simulink model "ECO_RM_WEC_EGEC"  (R2025a)
settings: Solver=ode4  StartTime=0  StopTime=120  FixedStep=0.00025  MaxStep=0.00025  RelTol=1e-3
values from neighbouring files (symbols this model uses):
  r = 0.043    [wecSimInputFile.m]
  simu = simulationClass()    [wecSimInputFile.m]
undefined symbols (not defined in the file or in its folder): body, constraint, DiscIntNeverNeededParam, geometry, hydroData, pto, ptoSim
libraries: WECSim_Lib_Body_Elements x2, WECSim_Lib_Frames x1, WECSim_Lib_Constraints x1, WECSim_Lib_PTOs x1
settings Model: Creator=pam1061  LastModifiedBy=pam1061
settings SolverCC: ZeroCrossControl=DisableAll  AutoInsertRateTranBlk=on
settings DataIOCC: ReturnWorkspaceOutputs=off
settings OptimizationCC: SimCompilerOptimization=on

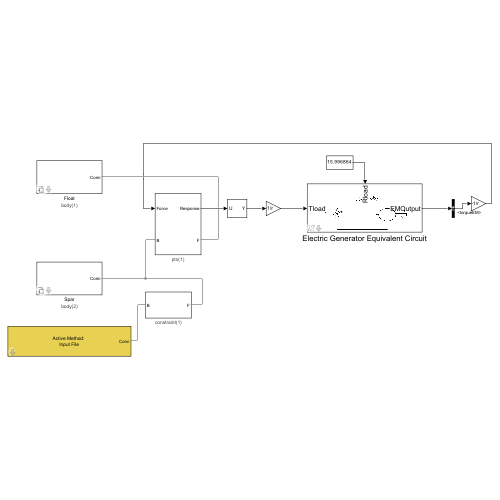
[thumbnail: Simulink's stored preview of the top-level diagram]
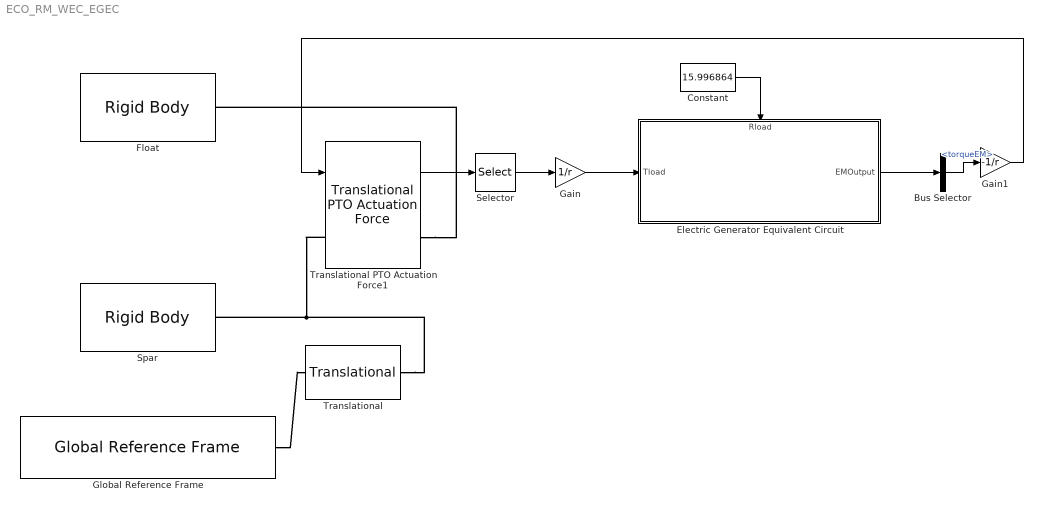
== system ECO_RM_WEC_EGEC ==
  Bus Selector : BusSelector  OutputSignals=torqueEM
  Constant : Constant  Value=15.996864
  Electric Generator Equivalent Circuit : Subsystem  AncestorBlock=WECSim_Lib_PTOSim/Electric/Electric Generator Equivalent Circuit  mask{ptoSim=ptoSim(1), InputFiletext=Use WEC-Sim input file to define Electric Machine parameters, Ra=0.890000, La=0.00500000, Ke=4.106198, bShaft=0, Jem=5.422000e-03}
      mask prompts: ptoSim "Electric Machine Name"; Ra "Armature Resistance [ohm]"; La "Armature Inductance [H]"; Ke "Back-emf or Torque constant [V/(rad/s)]"; bShaft "Rotor Damping [N s/m]"; Jem "Rotor Inertia [kg m^2]"
      mask init:
      | if exist('ptoSim','var')
      |     h=[gcb '/To Workspace'];
      |     responseName=['ptoSim' num2str(ptoSim.number) '_out'];
      |     set_param(h,'VariableName',responseName);
      | end
      | clear h responseName
      settings: PortSchema="{\"entries\":[{\"content\":{\"sides\":[{\"content\":{\"connectorIds\":[\"In1\"]},\"type\":\"ConnectorPlacement.EquallySpacedRectSide\",\"uuid\":\"38b15b7d-d952-45b6-9eb0-5d473736364e\"},{\"content\":{\"connectorIds\":[\"Out1\"],\"side\":\"RIGHT\"},\"type\":\"ConnectorPlacement.EquallySpacedRectSide\",\"uuid\":\"de64adb9-f2de-4dd5-b519-c63af884483d\"},{\"content\":{\"connectorIds\":[\"In2\"],\"side\":\"TOP\"},\"type\":\"ConnectorPlacement.EquallySpacedRectSide\",\"uuid\":\"eaa9506a-5e37-41b4-975c-a8d526700d36\"},{\"content\":{\"connectorIds\":[],\"side\":\"HIDDEN\"},\"type\":\"ConnectorPlacement.EquallySpacedRectSide\",\"uuid\":\"f8da1221-e5bc-4844-b966-beaaa1d6bf60\"}]},\"type\":\"ConnectorPlacement.EquallySpacedConnector\",\"uuid\":\"4da2b473-e94d-42dc-9143-64fbcbf5d9e1\"}],\"packageUris\":[\"http://schema.mathworks.com/mf0/Connector/R2020b\"],\"version\":\"1.0\"}"
      mask DialogControl CustomParameterGroup Prompt: Custom Parameters
      mask DialogControl EMParameters Prompt: Electric Machine Parameters
      mask Display: image('ElectricMotor.png'); % Use "Edit Image" on toolstrip to change.
  Float : WECSim_Lib_Body_Elements/Rigid Body  body=body(1)  h5File=hydroData/*.h5  geometryFile=geometry/*.stl  mass=0  inertia=0 0 0  inertiaProducts=0 0 0  nonHydro=0  nonlinearHydro=0  centerGravity=0 0 0  centerBuoyancy=0 0 0  dof=6  volume=0  displacement=0 0 0  axis=0 1 0  angle=0  option=0  cd=0 0 0  ca=0 0 0  area=0 0 0  VME=0  rgME=0 0 0  z=0 0 1
  Gain : Gain  Gain=1/r
  Gain1 : Gain  Gain=-1/r
  Global Reference Frame : WECSim_Lib_Frames/Global Reference Frame  waves=waves  simu=simu  InputMethod=Input File  InputFile=wecSimInputFile.m  mode=normal  explorer=off  solver=ode4  startTime=0  rampTime=100  endTime=400  dt=0.1  cicEndTime=60  stateSpace=0  WaveClass=regular  height=2.5  period=8  elevationFile=NOT DEFINED  spectrumFile=NOT DEFINED  direction=0  spread=1  spectrumType=NOT DEFINED  phaseSeed=0  option=EqualEnergy
  Selector : Selector  InputPortWidth=18  IndexOptions=Index vector (dialog)  Indices=9  OutputSizes=1
  Spar : WECSim_Lib_Body_Elements/Rigid Body  body=body(2)  h5File=hydroData/*.h5  geometryFile=geometry/*.stl  mass=0  inertia=0 0 0  inertiaProducts=0 0 0  nonHydro=0  nonlinearHydro=0  centerGravity=0 0 0  centerBuoyancy=0 0 0  dof=6  volume=0  displacement=0 0 0  axis=0 1 0  angle=0  option=0  cd=0 0 0  ca=0 0 0  area=0 0 0  VME=0  rgME=0 0 0  z=0 0 1
  Translational : WECSim_Lib_Constraints/Translational  constraint=constraint(1)  loc="0  0  0"  displacement=0 0 0  y=0 1 0  z=0 0 1  upperLimitSpecify=off  upperLimitBound=0  upperLimitTransitionRegionWidth=0  upperLimitStiffness=0  upperLimitDamping=0  lowerLimitSpecify=off  lowerLimitBound=0  lowerLimitTransitionRegionWidth=0  lowerLimitStiffness=0  lowerLimitDamping=0
      settings: AttributesFormatString=%<constraint>
  Translational PTO Actuation Force1 : WECSim_Lib_PTOs/Translational PTO Actuation Force  pto=pto(1)  loc="0  0  0"  stiffness=0  damping=0  equilibriumPosition=0  pretension=0  displacement=0 0 0  y=0 1 0  z=0 0 1  upperLimitSpecify=off  upperLimitBound=0  upperLimitTransitionRegionWidth=0  upperLimitStiffness=0  upperLimitDamping=0  lowerLimitSpecify=off  lowerLimitBound=0  lowerLimitTransitionRegionWidth=0  lowerLimitStiffness=0  lowerLimitDamping=0
      settings: AttributesFormatString=%<pto>
  wires:
  Translational PTO Actuation Force1/1 -> Selector/1
  Gain1/1 -> Translational PTO Actuation Force1/1
  Constant/1 -> Electric Generator Equivalent Circuit/2(Rload)
  Selector/1 -> Gain/1
  Gain/1 -> Electric Generator Equivalent Circuit/1(Tload)
  Electric Generator Equivalent Circuit/1(EMOutput) -> Bus Selector/1
  Bus Selector/1 -> Gain1/1  "<torqueEM>"
  connections:
  Global Reference Frame/RConn1 -- Translational/LConn1
  Translational/RConn1 -- Translational PTO Actuation Force1/LConn1 -- Spar/RConn1
  Translational PTO Actuation Force1/RConn1 -- Float/RConn1

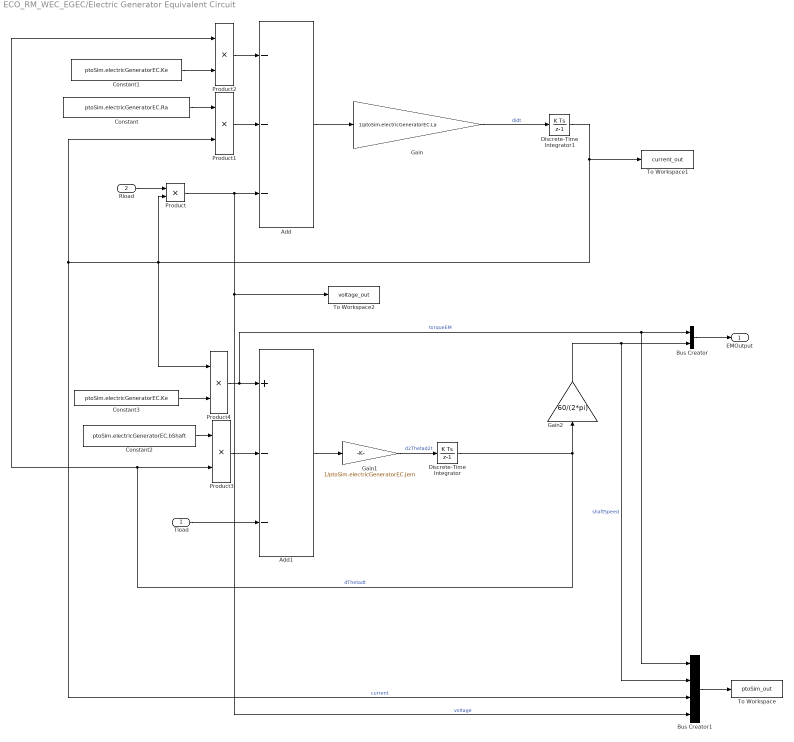
== system ECO_RM_WEC_EGEC/Electric Generator Equivalent Circuit ==
  Tload : Inport
  Rload : Inport  Port=2
  Add : Sum  Inputs=---
  Add1 : Sum  Inputs=+--
  Bus Creator : BusCreator  Inputs=2
  Bus Creator1 : BusCreator  Inputs=4
  Constant : Constant  Value=ptoSim.electricGeneratorEC.Ra
  Constant1 : Constant  Value=ptoSim.electricGeneratorEC.Ke
  Constant2 : Constant  Value=ptoSim.electricGeneratorEC.bShaft
  Constant3 : Constant  Value=ptoSim.electricGeneratorEC.Ke
  Discrete-Time Integrator : DiscreteIntegrator  InitialCondition=(2*pi/60)*ptoSim.electricGeneratorEC.wShaftIni  SampleTime=-1  ICPrevOutput=DiscIntNeverNeededParam  ICPrevScaledInput=DiscIntNeverNeededParam
  Discrete-Time Integrator1 : DiscreteIntegrator  InitialCondition=ptoSim.electricGeneratorEC.currentIni  SampleTime=-1  ICPrevOutput=DiscIntNeverNeededParam  ICPrevScaledInput=DiscIntNeverNeededParam
  Gain : Gain  Gain=1/ptoSim.electricGeneratorEC.La
  Gain1 : Gain  Gain=1/ptoSim.electricGeneratorEC.Jem
  Gain2 : Gain  Gain=60/(2*pi)
  Product{,1..4} (5 alike) : Product
  To Workspace : ToWorkspace  VariableName=ptoSim_out  SaveFormat=Structure With Time  SampleTime=simu.dtOut
  To Workspace1 : ToWorkspace  VariableName=current_out  SampleTime=-1
  To Workspace2 : ToWorkspace  VariableName=voltage_out  SampleTime=-1
  EMOutput : Outport
  wires:
  Bus Creator1/1 -> To Workspace/1
  Gain2/1 -> Bus Creator/2, Bus Creator1/2  "shaftSpeed"
  Bus Creator/1 -> EMOutput/1
  Constant3/1 -> Product4/2
  Product4/1 -> Add1/1, Bus Creator/1, Bus Creator1/1  "torqueEM"
  Discrete-Time Integrator/1 -> Gain2/1, Product3/2, Product2/1  "dThetadt"
  Constant2/1 -> Product3/1
  Product3/1 -> Add1/2
  Gain1/1 -> Discrete-Time Integrator/1  "d2Thetad2t"
  Add1/1 -> Gain1/1
  Tload/1 -> Add1/3
  Constant1/1 -> Product2/2
  Product2/1 -> Add/1
  Constant/1 -> Product1/1
  Product1/1 -> Add/2
  Product/1 -> Add/3, To Workspace2/1, Bus Creator1/4  "voltage"
  Discrete-Time Integrator1/1 -> To Workspace1/1, Product1/2, Bus Creator1/3, Product/2, Product4/1  "current"
  Rload/1 -> Product/1
  Gain/1 -> Discrete-Time Integrator1/1  "didt"
  Add/1 -> Gain/1
